simulink model "EX002_FCHEV"  (R2020b)
settings: Solver=ode23tb  StartTime=0.0  StopTime=20e3  MaxStep=1  RelTol=1e-3
libraries: component_lib x27, pid_lib x3
settings Model: Creator=maxjo65  LastModifiedBy=Max

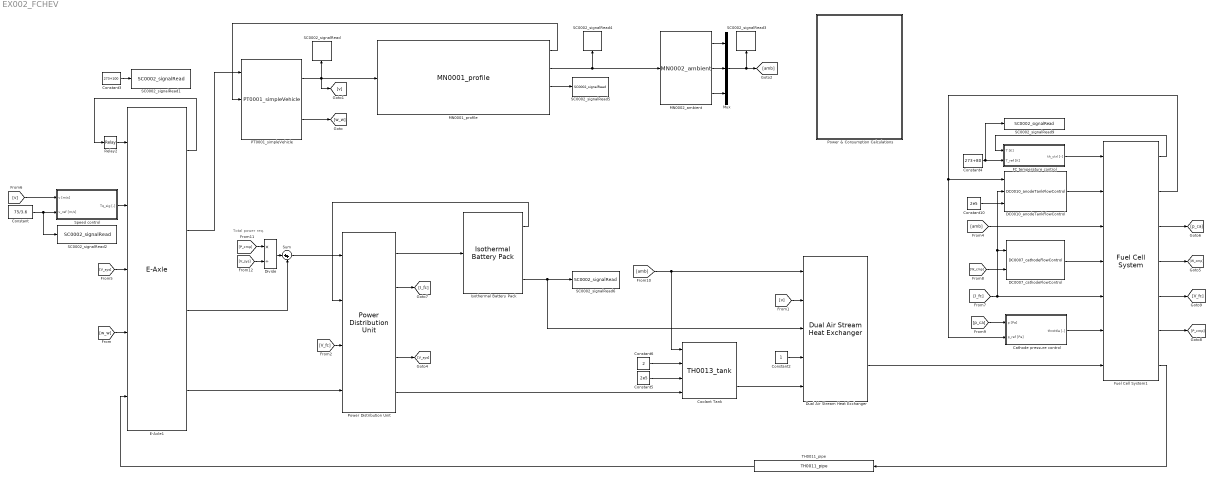
== system EX002_FCHEV ==
  note: Total power req.
  Cathode pressure control : Subsystem
  Constant : Constant  Value=75/3.6
  Constant10 : Constant  Value=2e5
  Constant2 : Constant
  Constant3 : Constant  Value=273+100
  Constant4 : Constant  Value=273+80
  Constant5 : Constant  Value=2e5
  Constant6 : Constant  Value=2
  Coolant Tank : component_lib/Thermal Systems/TH0013_tank  V=5e-3
  DC0007_cathodeFlowControl : component_lib/Data & Control/DC0007_cathodeFlowControl  lambda_O2_ref=2  n_cell=335
  DC0010_anodeTankFlowControl : component_lib/Data & Control/DC0010_anodeTankFlowControl  n_cell=335
  Divide : Product  Inputs=*/
  Dual Air Stream Heat Exchanger : component_lib/Dual Air Stream Heat Exchanger  HtH=1.1  StS=0.95
  E-Axle1 : component_lib/E-Axle  n=2
  FC temperature control : Subsystem
  Fuel Cell System1 : component_lib/Fuel Cell System  n_st=2
  Isothermal Battery Pack : component_lib/Isothermal Battery Pack  SOC_0=0.5  n_mod_ser=16  n_mod_par=1  T=273+25
  MN0001_profile : component_lib/Mission/MN0001_profile  profile=KoblenzTrier.mat  x0=0  N_lookahead=100
  MN0002_ambient : component_lib/Mission/MN0002_ambient  p_0=1.01e5  T_0=273 + 20  RH_0=0.2
  Mux : Mux  Inputs=3
  PT0001_simpleVehicle : component_lib/Powertrain/PT0001_simpleVehicle  m=40e3  r_w=0.5  A_f=10  C_d=0.5  rho_air=1.225  c_r0=0.0060  c_r1=2.3e-7  gain=600  v0=75/3.6  x0=0
  Power & Consumption Calculations : Subsystem
  Power Distribution Unit : component_lib/Power Distribution Unit  V_sys=420  P_fc=80e3  I_bt_max=350  I_bt_min=-200  T_s=5
  Relay2 : Relay  OnSwitchValue=373+5  OffSwitchValue=373-5
  SC0002_signalRead : component_lib/Data & Control/SC0002_signalRead  SigName=velocity
  SC0002_signalRead1 : component_lib/Data & Control/SC0002_signalRead  SigName=motorTemperatureReference
  SC0002_signalRead2 : component_lib/Data & Control/SC0002_signalRead  SigName=velocityReference
  SC0002_signalRead3 : component_lib/Data & Control/SC0002_signalRead  SigName=ambient
  SC0002_signalRead4 : component_lib/Data & Control/SC0002_signalRead  SigName=altitude
  SC0002_signalRead5 : component_lib/Data & Control/SC0002_signalRead  SigName=distance
  SC0002_signalRead6 : component_lib/Data & Control/SC0002_signalRead  SigName=batteryHeatingPower
  SC0002_signalRead9 : component_lib/Data & Control/SC0002_signalRead  SigName=fuelCellTemperatureReference
  Speed control : Subsystem
  Sum : Sum  Inputs=|++
  TH0011_pipe : component_lib/Thermal Systems/TH0011_pipe  d=3e-2  L=2  T_0=273 + 20  p_0=2e5  W_0=2
  wires:
  MN0001_profile/2 -> MN0002_ambient/1, SC0002_signalRead4/1
  Constant/1 -> Speed control/2(v_ref [m/s]), SC0002_signalRead2/1
  PT0001_simpleVehicle/1 -> SC0002_signalRead/1, [v], MN0001_profile/1
  PT0001_simpleVehicle/2 -> [w_w]
  MN0001_profile/1 -> PT0001_simpleVehicle/2
  [V_fc] -> Power Distribution Unit/3
  TH0011_pipe/1 -> E-Axle1/5
  Dual Air Stream Heat Exchanger/2 -> Fuel Cell System1/7
  Mux/1 -> [amb], SC0002_signalRead3/1
  [amb] -> Coolant Tank/1, Dual Air Stream Heat Exchanger/1
  MN0002_ambient/2 -> Mux/2
  MN0002_ambient/1 -> Mux/1
  MN0002_ambient/3 -> Mux/3
  Isothermal Battery Pack/1 -> Power Distribution Unit/2
  E-Axle1/4 -> Power Distribution Unit/4
  Power Distribution Unit/2 -> [I_fc]
  Power Distribution Unit/4 -> [V_sys]
  Power Distribution Unit/5 -> Coolant Tank/4
  MN0001_profile/3 -> SC0002_signalRead5/1
  Coolant Tank/2 -> Dual Air Stream Heat Exchanger/5
  Constant5/1 -> Coolant Tank/3
  Constant6/1 -> Coolant Tank/2
  Constant4/1 -> SC0002_signalRead9/1, FC temperature control/2(T_ref [K])
  Power Distribution Unit/1 -> Isothermal Battery Pack/1
  [V_sys] -> E-Axle1/3
  [w_w] -> E-Axle1/4
  Speed control/1(Tq_sig [-]) -> E-Axle1/2
  E-Axle1/2 -> PT0001_simpleVehicle/1
  [v] -> Speed control/1(v [m/s])
  Constant3/1 -> SC0002_signalRead1/1
  Relay2/1 -> E-Axle1/1
  E-Axle1/1 -> Relay2/1
  [v] -> Dual Air Stream Heat Exchanger/2
  [I_fc] -> DC0007_cathodeFlowControl/1, DC0010_anodeTankFlowControl/2, Fuel Cell System1/5
  [amb] -> Fuel Cell System1/3
  DC0010_anodeTankFlowControl/1 -> Fuel Cell System1/2
  Fuel Cell System1/7 -> TH0011_pipe/1
  DC0007_cathodeFlowControl/1 -> Fuel Cell System1/4
  Cathode pressure control/1(throttle [-]) -> Fuel Cell System1/6
  Constant10/1 -> DC0010_anodeTankFlowControl/3
  Fuel Cell System1/5 -> [V_fc]
  Fuel Cell System1/4 -> [W_cmp]
  [W_cmp] -> DC0007_cathodeFlowControl/2
  Fuel Cell System1/3 -> [p_ca]
  [p_ca] -> Cathode pressure control/1(p [Pa])
  FC temperature control/1(th_ctrl [-]) -> Fuel Cell System1/1
  Fuel Cell System1/1 -> FC temperature control/1(T [K])
  Fuel Cell System1/6 -> [P_cmp]
  Sum/1 -> Power Distribution Unit/1
  [P_cmp] -> Divide/1
  [V_sys] -> Divide/2
  Divide/1 -> Sum/1
  E-Axle1/3 -> Sum/2
  Fuel Cell System1/2 -> DC0010_anodeTankFlowControl/1, Cathode pressure control/2(p_ref [Pa])
  Constant2/1 -> Dual Air Stream Heat Exchanger/4
  Isothermal Battery Pack/3 -> Dual Air Stream Heat Exchanger/3, SC0002_signalRead6/1

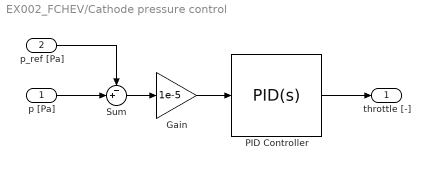
== system EX002_FCHEV/Cathode pressure control ==
  p [Pa] : Inport
  p_ref [Pa] : Inport  Port=2
  Gain : Gain  Gain=1e-5
  PID Controller : pid_lib/PID Controller  Controller=PID  Form=Parallel  TimeDomain=Continuous-time  UseExternalTs=off  SampleTime=-1  IntegratorMethod=Forward Euler  FilterMethod=Forward Euler  ControllerParametersSource=internal  P=1  I=0  D=0  UseFilter=on  N=100  TunerSelectOption=Transfer Function Based (PID Tuner App)  InitialConditionSource=internal  InitialConditionForIntegrator=0  InitialConditionForFilter=0  DifferentiatorICPrevScaledInput=0  ExternalReset=none  TrackingMode=off  Kt=1  LimitOutput=on  SatLimitsSource=internal  UpperSaturationLimit=1  LowerSaturationLimit=0  LinearizeAsGain=on  AntiWindupMode=clamping  Kb=1  POutMin=[]  POutMax=[]  IOutMin=[]  IOutMax=[]  DOutMin=[]  DOutMax=[]  NOutMin=[]  NOutMax=[]  SumOutMin=[]  SumOutMax=[]  SaturationOutMin=[]  SaturationOutMax=[]  PParamMin=[]  PParamMax=[]  IParamMin=[]  IParamMax=[]  DParamMin=[]  DParamMax=[]  NParamMin=[]  NParamMax=[]  KbParamMin=[]  KbParamMax=[]  KtParamMin=[]  KtParamMax=[]  KbOutMin=[]  KbOutMax=[]  KtOutMin=[]  KtOutMax=[]  IntegratorOutMin=[]  IntegratorOutMax=[]  FilterOutMin=[]  FilterOutMax=[]  SumI1OutMin=[]  SumI1OutMax=[]  SumI2OutMin=[]  SumI2OutMax=[]  SumI3OutMin=[]  SumI3OutMax=[]  SumI4OutMin=[]  SumI4OutMax=[]  SumDOutMin=[]  SumDOutMax=[]  DifferentiatorOutMin=[]  DifferentiatorOutMax=[]  FilterDiffOutCoefMin=[]  FilterDiffOutCoefMax=[]  ReciprocalOutMin=[]  ReciprocalOutMax=[]  SumDenOutMin=[]  SumDenOutMax=[]  SumNumOutMin=[]  SumNumOutMax=[]  DivideOutMin=[]  DivideOutMax=[]  UdiffTsProdOutMin=[]  UdiffTsProdOutMax=[]  NTsProdOutMin=[]  NTsProdOutMax=[]  UintegralTsProdOutMin=[]  UintegralTsProdOutMax=[]  UngainTsProdOutMin=[]  UngainTsProdOutMax=[]  IntegratorContinuousStateAttributes=''  IntegratorStateMustResolveToSignalObject=off  IntegratorRTWStateStorageClass=Auto  FilterContinuousStateAttributes=''  FilterStateMustResolveToSignalObject=off  FilterRTWStateStorageClass=Auto  ParallelPVariant=InternalParameters  IdealPVariant=Disabled  IVariant=InternalParameters  DVariant=InternalParameters  IntegratorVariant=Continuous  SatVariant=Enabled  AWVariant=ContClampingParallel  PCopyVariant=Disabled  TRVariant=Disabled  FdbkBlocksVariant=Forward  IdealPFdbkVariant=Disabled  SatFdbkVariant=Disabled  DerivativeFilterVariant=ContFilter  NVariant=InternalParameters  NCopyVariant=Disabled  FilterICVariant=InternalICsFilter  IntegratorICVariant=InternalICs  ExternalResetVariant=Disabled  TRSumVariant=Passthrough  SumFdbkVariant=Disabled  SumVariant=Sum_PID  TsampFilterVariant=InternalTs  TsampNgainVariant=Passthrough  TsampIntegralVariant=Passthrough  ExternalSaturationOutDataTypeStr=Inherit: Same as second input
  Sum : Sum  Inputs=-+|
  throttle [-] : Outport
  wires:
  PID Controller/1 -> throttle [-]/1
  p_ref [Pa]/1 -> Sum/1
  p [Pa]/1 -> Sum/2
  Sum/1 -> Gain/1
  Gain/1 -> PID Controller/1

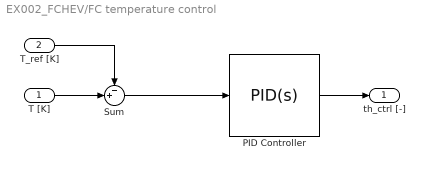
== system EX002_FCHEV/FC temperature control ==
  T [K] : Inport
  T_ref [K] : Inport  Port=2
  PID Controller : pid_lib/PID Controller  Controller=PID  Form=Parallel  TimeDomain=Continuous-time  UseExternalTs=off  SampleTime=-1  IntegratorMethod=Forward Euler  FilterMethod=Forward Euler  ControllerParametersSource=internal  P=1e-2  I=1e-3  D=0  UseFilter=on  N=100  TunerSelectOption=Transfer Function Based (PID Tuner App)  InitialConditionSource=internal  InitialConditionForIntegrator=0  InitialConditionForFilter=0  DifferentiatorICPrevScaledInput=0  ExternalReset=none  TrackingMode=off  Kt=1  LimitOutput=on  SatLimitsSource=internal  UpperSaturationLimit=1  LowerSaturationLimit=0  LinearizeAsGain=on  AntiWindupMode=clamping  Kb=1  POutMin=[]  POutMax=[]  IOutMin=[]  IOutMax=[]  DOutMin=[]  DOutMax=[]  NOutMin=[]  NOutMax=[]  SumOutMin=[]  SumOutMax=[]  SaturationOutMin=[]  SaturationOutMax=[]  PParamMin=[]  PParamMax=[]  IParamMin=[]  IParamMax=[]  DParamMin=[]  DParamMax=[]  NParamMin=[]  NParamMax=[]  KbParamMin=[]  KbParamMax=[]  KtParamMin=[]  KtParamMax=[]  KbOutMin=[]  KbOutMax=[]  KtOutMin=[]  KtOutMax=[]  IntegratorOutMin=[]  IntegratorOutMax=[]  FilterOutMin=[]  FilterOutMax=[]  SumI1OutMin=[]  SumI1OutMax=[]  SumI2OutMin=[]  SumI2OutMax=[]  SumI3OutMin=[]  SumI3OutMax=[]  SumI4OutMin=[]  SumI4OutMax=[]  SumDOutMin=[]  SumDOutMax=[]  DifferentiatorOutMin=[]  DifferentiatorOutMax=[]  FilterDiffOutCoefMin=[]  FilterDiffOutCoefMax=[]  ReciprocalOutMin=[]  ReciprocalOutMax=[]  SumDenOutMin=[]  SumDenOutMax=[]  SumNumOutMin=[]  SumNumOutMax=[]  DivideOutMin=[]  DivideOutMax=[]  UdiffTsProdOutMin=[]  UdiffTsProdOutMax=[]  NTsProdOutMin=[]  NTsProdOutMax=[]  UintegralTsProdOutMin=[]  UintegralTsProdOutMax=[]  UngainTsProdOutMin=[]  UngainTsProdOutMax=[]  IntegratorContinuousStateAttributes=''  IntegratorStateMustResolveToSignalObject=off  IntegratorRTWStateStorageClass=Auto  FilterContinuousStateAttributes=''  FilterStateMustResolveToSignalObject=off  FilterRTWStateStorageClass=Auto  ParallelPVariant=InternalParameters  IdealPVariant=Disabled  IVariant=InternalParameters  DVariant=InternalParameters  IntegratorVariant=Continuous  SatVariant=Enabled  AWVariant=ContClampingParallel  PCopyVariant=Disabled  TRVariant=Disabled  FdbkBlocksVariant=Forward  IdealPFdbkVariant=Disabled  SatFdbkVariant=Disabled  DerivativeFilterVariant=ContFilter  NVariant=InternalParameters  NCopyVariant=Disabled  FilterICVariant=InternalICsFilter  IntegratorICVariant=InternalICs  ExternalResetVariant=Disabled  TRSumVariant=Passthrough  SumFdbkVariant=Disabled  SumVariant=Sum_PID  TsampFilterVariant=InternalTs  TsampNgainVariant=Passthrough  TsampIntegralVariant=Passthrough  ExternalSaturationOutDataTypeStr=Inherit: Same as second input
  Sum : Sum  Inputs=-+|
  th_ctrl [-] : Outport
  wires:
  PID Controller/1 -> th_ctrl [-]/1
  T_ref [K]/1 -> Sum/1
  T [K]/1 -> Sum/2
  Sum/1 -> PID Controller/1

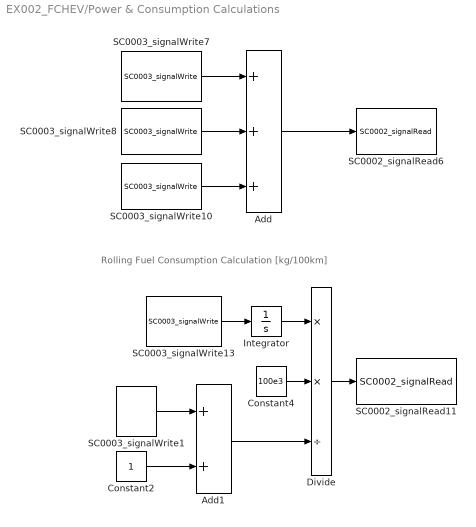
== system EX002_FCHEV/Power & Consumption Calculations ==
  note: Rolling Fuel Consumption Calculation [kg/100km]
  Add : Sum  Inputs=+++
  Add1 : Sum
  Constant2 : Constant
  Constant4 : Constant  Value=100e3
  Divide : Product  Inputs=**/
  Integrator : Integrator
  SC0002_signalRead11 : component_lib/Data & Control/SC0002_signalRead  SigName=fuelConsumption
  SC0002_signalRead6 : component_lib/Data & Control/SC0002_signalRead  SigName=producedPower
  SC0003_signalWrite1 : component_lib/Data & Control/SC0003_signalWrite  SigName=distance
  SC0003_signalWrite10 : component_lib/Data & Control/SC0003_signalWrite  SigName=burnOffPower
  SC0003_signalWrite13 : component_lib/Data & Control/SC0003_signalWrite  SigName=hydrogenFlow
  SC0003_signalWrite7 : component_lib/Data & Control/SC0003_signalWrite  SigName=batteryPower
  SC0003_signalWrite8 : component_lib/Data & Control/SC0003_signalWrite  SigName=fuelCellPower
  wires:
  Integrator/1 -> Divide/1
  SC0003_signalWrite7/1 -> Add/1
  SC0003_signalWrite10/1 -> Add/3
  SC0003_signalWrite1/1 -> Add1/1
  SC0003_signalWrite8/1 -> Add/2
  Add/1 -> SC0002_signalRead6/1
  Add1/1 -> Divide/3
  Constant4/1 -> Divide/2
  Constant2/1 -> Add1/2
  Divide/1 -> SC0002_signalRead11/1
  SC0003_signalWrite13/1 -> Integrator/1

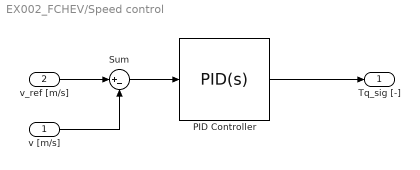
== system EX002_FCHEV/Speed control ==
  v [m/s] : Inport
  v_ref [m/s] : Inport  Port=2
  PID Controller : pid_lib/PID Controller  Controller=PID  Form=Parallel  TimeDomain=Continuous-time  UseExternalTs=off  SampleTime=-1  IntegratorMethod=Forward Euler  FilterMethod=Forward Euler  ControllerParametersSource=internal  P=10  I=1e-1  D=0  UseFilter=on  N=100  TunerSelectOption=Transfer Function Based (PID Tuner App)  InitialConditionSource=internal  InitialConditionForIntegrator=0  InitialConditionForFilter=0  DifferentiatorICPrevScaledInput=0  ExternalReset=none  TrackingMode=off  Kt=1  LimitOutput=on  SatLimitsSource=internal  UpperSaturationLimit=1  LowerSaturationLimit=-1  LinearizeAsGain=on  AntiWindupMode=clamping  Kb=1  POutMin=[]  POutMax=[]  IOutMin=[]  IOutMax=[]  DOutMin=[]  DOutMax=[]  NOutMin=[]  NOutMax=[]  SumOutMin=[]  SumOutMax=[]  SaturationOutMin=[]  SaturationOutMax=[]  PParamMin=[]  PParamMax=[]  IParamMin=[]  IParamMax=[]  DParamMin=[]  DParamMax=[]  NParamMin=[]  NParamMax=[]  KbParamMin=[]  KbParamMax=[]  KtParamMin=[]  KtParamMax=[]  KbOutMin=[]  KbOutMax=[]  KtOutMin=[]  KtOutMax=[]  IntegratorOutMin=[]  IntegratorOutMax=[]  FilterOutMin=[]  FilterOutMax=[]  SumI1OutMin=[]  SumI1OutMax=[]  SumI2OutMin=[]  SumI2OutMax=[]  SumI3OutMin=[]  SumI3OutMax=[]  SumI4OutMin=[]  SumI4OutMax=[]  SumDOutMin=[]  SumDOutMax=[]  DifferentiatorOutMin=[]  DifferentiatorOutMax=[]  FilterDiffOutCoefMin=[]  FilterDiffOutCoefMax=[]  ReciprocalOutMin=[]  ReciprocalOutMax=[]  SumDenOutMin=[]  SumDenOutMax=[]  SumNumOutMin=[]  SumNumOutMax=[]  DivideOutMin=[]  DivideOutMax=[]  UdiffTsProdOutMin=[]  UdiffTsProdOutMax=[]  NTsProdOutMin=[]  NTsProdOutMax=[]  UintegralTsProdOutMin=[]  UintegralTsProdOutMax=[]  UngainTsProdOutMin=[]  UngainTsProdOutMax=[]  IntegratorContinuousStateAttributes=''  IntegratorStateMustResolveToSignalObject=off  IntegratorRTWStateStorageClass=Auto  FilterContinuousStateAttributes=''  FilterStateMustResolveToSignalObject=off  FilterRTWStateStorageClass=Auto  ParallelPVariant=InternalParameters  IdealPVariant=Disabled  IVariant=InternalParameters  DVariant=InternalParameters  IntegratorVariant=Continuous  SatVariant=Enabled  AWVariant=ContClampingParallel  PCopyVariant=Disabled  TRVariant=Disabled  FdbkBlocksVariant=Forward  IdealPFdbkVariant=Disabled  SatFdbkVariant=Disabled  DerivativeFilterVariant=ContFilter  NVariant=InternalParameters  NCopyVariant=Disabled  FilterICVariant=InternalICsFilter  IntegratorICVariant=InternalICs  ExternalResetVariant=Disabled  TRSumVariant=Passthrough  SumFdbkVariant=Disabled  SumVariant=Sum_PID  TsampFilterVariant=InternalTs  TsampNgainVariant=Passthrough  TsampIntegralVariant=Passthrough  ExternalSaturationOutDataTypeStr=Inherit: Same as second input
  Sum : Sum  Inputs=|+-
  Tq_sig [-] : Outport
  wires:
  PID Controller/1 -> Tq_sig [-]/1
  Sum/1 -> PID Controller/1
  v_ref [m/s]/1 -> Sum/1
  v [m/s]/1 -> Sum/2
